simulink model "refricyc"  (R2015a)
settings: Solver=ode45  StartTime=0.0  StopTime=10.0  RelTol=1e-3
libraries: simulink x2
settings Model: Creator=Mabele  LastModifiedBy=Mabele

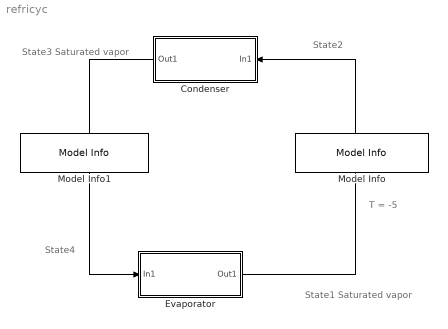
== system refricyc ==
  note: T = -5
  note: State4
  note: State2
  note: State3
      | Saturated vapor
  note: State1
      | Saturated vapor
  Condenser : Subsystem
  Evaporator : Subsystem
  Model Info : simulink/Model-Wide Utilities/Model Info  Frame=on  DisplayStringWithTags=Compressor  HorizontalTextAlignment=Center  LeftAlignmentValue=0.5  SourceBlockDiagram=refricyc  TagMaxNumber=20
  Model Info1 : simulink/Model-Wide Utilities/Model Info  Frame=on  DisplayStringWithTags=Throttle/Expansion valve  HorizontalTextAlignment=Center  LeftAlignmentValue=0.5  SourceBlockDiagram=refricyc  TagMaxNumber=20
  wires:
  Condenser/1(Out1) -> Evaporator/1(In1)
  Evaporator/1(Out1) -> Condenser/1(In1)

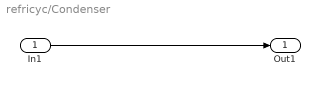
== system refricyc/Condenser ==
  In1 : Inport
  Out1 : Outport
  wires:
  In1/1 -> Out1/1

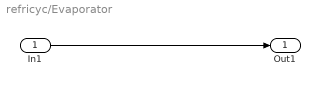
== system refricyc/Evaporator ==
  In1 : Inport
  Out1 : Outport
  wires:
  In1/1 -> Out1/1
